simulink library "courseFollow_cl"  (R2018b)
settings: Solver=VariableStepAuto  StartTime=0.0  StopTime=10.0  RelTol=1e-3
undefined symbols (not defined in the file): a, initS, pathCtrl
libraries: angleBtw2Vecs_ul x3, vectorNormalizer_ul x3, schmehlTangentRotation_ul x1
settings Model: Creator=James Reed  LastModifiedBy=mcobb

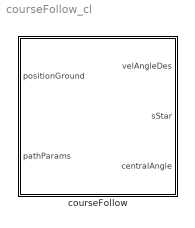
== system courseFollow_cl ==
  courseFollow : Subsystem

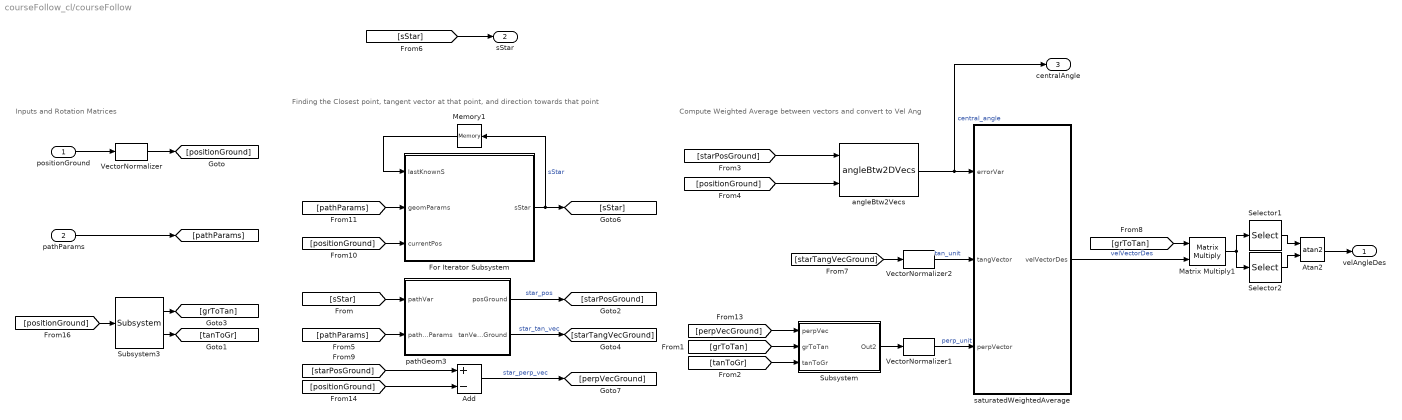
== system courseFollow_cl/courseFollow ==
  note: Compute Weighted Average between vectors and convert to Vel Ang
  note: Inputs and Rotation Matrices
  note: Finding the Closest point, tangent vector at that point, and direction towards that point
  "positionGround " : Inport
  pathParams : Inport  Port=2
  Add : Sum  Inputs=+-
  Atan2 : Trigonometry  Operator=atan2
  For Iterator Subsystem : Subsystem  TreatAsAtomicUnit=on
  Matrix Multiply1 : Product  Multiplication=Matrix(*)
  Memory1 : Memory  InitialCondition=initS
  Selector1 : Selector  InputPortWidth=3  IndexOptions=Index vector (dialog)  Indices=2  OutputSizes=1
  Selector2 : Selector  InputPortWidth=3  IndexOptions=Index vector (dialog)  Indices=1  OutputSizes=1
  Subsystem : Subsystem
  Subsystem3 : schmehlTangentRotation_ul/Subsystem  SystemSampleTime=-1
  "VectorNormalizer " : vectorNormalizer_ul/VectorNormalizer   SystemSampleTime=-1
  VectorNormalizer1 : vectorNormalizer_ul/VectorNormalizer   SystemSampleTime=-1
  VectorNormalizer2 : vectorNormalizer_ul/VectorNormalizer   SystemSampleTime=-1
  angleBtw2Vecs : angleBtw2Vecs_ul/angleBtw2DVecs  SystemSampleTime=-1
  pathGeom3 : MATLAB Function  TreatAsAtomicUnit=on
  saturatedWeightedAverage : Subsystem  mask{error_upper_lim=pathCtrl.perpErrorVal.Value}
      mask prompts: error_upper_lim "Value of Error yielding 100% perpendicular"
  velAngleDes : Outport
  sStar : Outport  Port=2
  centralAngle : Outport  Port=3
  wires:
  "VectorNormalizer "/1 -> [positionGround]
  [starPosGround] -> angleBtw2Vecs/1
  pathParams/1 -> [pathParams]
  VectorNormalizer2/1 -> saturatedWeightedAverage/2(tangVector)  "tan_unit"
  saturatedWeightedAverage/1("velVectorDes ") -> Matrix Multiply1/2  "velVectorDes"
  [positionGround] -> For Iterator Subsystem/3(currentPos)
  [positionGround] -> Subsystem3/1
  "positionGround "/1 -> "VectorNormalizer "/1
  Subsystem3/1 -> [grToTan]
  pathGeom3/1(posGround) -> [starPosGround]  "star_pos"
  [pathParams] -> pathGeom3/2(pathGeomParams)
  VectorNormalizer1/1 -> saturatedWeightedAverage/3("perpVector ")  "perp_unit"
  angleBtw2Vecs/1 -> centralAngle/1, saturatedWeightedAverage/1("errorVar ")  "central_angle"
  [positionGround] -> angleBtw2Vecs/2
  [sStar] -> pathGeom3/1(pathVar)
  [starTangVecGround] -> VectorNormalizer2/1
  [pathParams] -> For Iterator Subsystem/2(geomParams)
  Subsystem3/2 -> [tanToGr]
  [grToTan] -> Matrix Multiply1/1
  Matrix Multiply1/1 -> Selector2/1, Selector1/1
  Selector1/1 -> Atan2/1
  Selector2/1 -> Atan2/2
  Atan2/1 -> velAngleDes/1
  For Iterator Subsystem/1(sStar) -> [sStar], Memory1/1  "sStar"
  Memory1/1 -> For Iterator Subsystem/1(lastKnownS)
  Add/1 -> [perpVecGround]  "star_perp_vec"
  [positionGround] -> Add/2
  [starPosGround] -> Add/1
  pathGeom3/2(tanVecGround) -> [starTangVecGround]  "star_tan_vec"
  [perpVecGround] -> Subsystem/1(perpVec)
  Subsystem/1(Out2) -> VectorNormalizer1/1
  [grToTan] -> Subsystem/2(grToTan)
  [tanToGr] -> Subsystem/3(tanToGr)
  [sStar] -> sStar/1

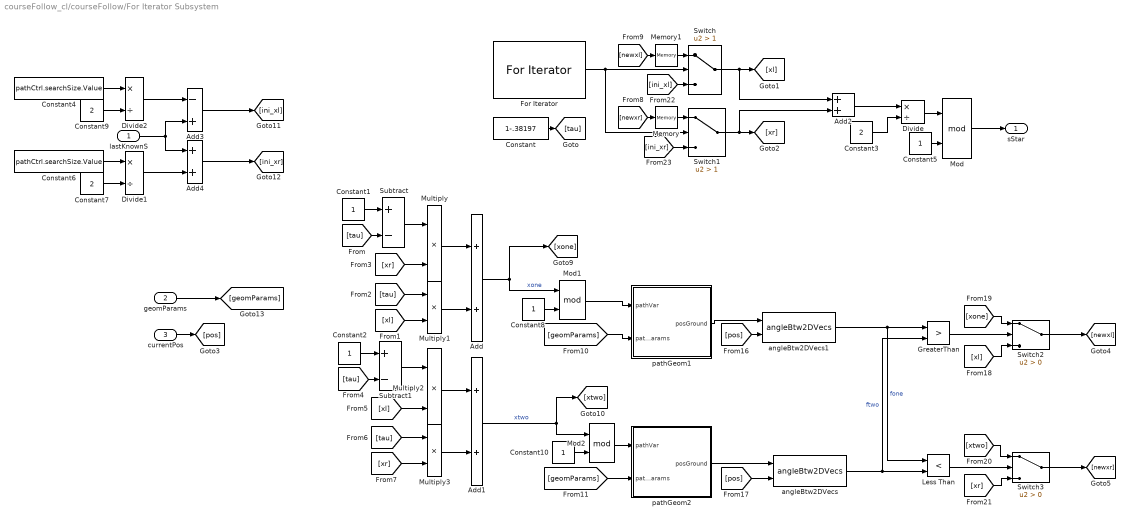
== system courseFollow_cl/courseFollow/For Iterator Subsystem ==
  lastKnownS : Inport
  geomParams : Inport  Port=2
  currentPos : Inport  Port=3
  Add{,1..2,4} (4 alike) : Sum
  Add3 : Sum  Inputs=-+
  Constant : Constant  Value=1-.38197
  Constant{1..2,5,8,10} (5 alike) : Constant
  Constant3 : Constant  Value=2
  Constant4 : Constant  Value=pathCtrl.searchSize.Value
  Constant6 : Constant  Value=pathCtrl.searchSize.Value
  Constant7 : Constant  Value=2
  Constant9 : Constant  Value=2
  Divide : Product  Inputs=*/
  Divide1 : Product  Inputs=*/
  Divide2 : Product  Inputs=*/
  For Iterator : ForIterator  IterationLimit=100
  GreaterThan : RelationalOperator  Operator=>  OutDataTypeStr=boolean  RndMeth=Simplest
  Less Than : RelationalOperator  Operator=<  OutDataTypeStr=boolean  RndMeth=Simplest
  Memory : Memory  InheritSampleTime=on
  Memory1 : Memory  InheritSampleTime=on
  Mod : Math  Operator=mod  SaturateOnIntegerOverflow=on
  Mod1 : Math  Operator=mod  SaturateOnIntegerOverflow=on
  Mod2 : Math  Operator=mod  SaturateOnIntegerOverflow=on
  Multiply{,1..3} (4 alike) : Product
  Subtract : Sum  Inputs=+-
  Subtract1 : Sum  Inputs=+-
  Switch : Switch  Criteria=u2 > Threshold  Threshold=1
  Switch1 : Switch  Criteria=u2 > Threshold  Threshold=1
  Switch2 : Switch  Criteria=u2 > Threshold
  Switch3 : Switch  Criteria=u2 > Threshold
  angleBtw2DVecs : angleBtw2Vecs_ul/angleBtw2DVecs  SystemSampleTime=-1
  angleBtw2DVecs1 : angleBtw2Vecs_ul/angleBtw2DVecs  SystemSampleTime=-1
  pathGeom1 : MATLAB Function  TreatAsAtomicUnit=on
  pathGeom2 : MATLAB Function  TreatAsAtomicUnit=on
  sStar : Outport
  wires:
  Constant3/1 -> Divide/2
  Add2/1 -> Divide/1
  Constant/1 -> [tau]
  Constant1/1 -> Subtract/1
  [tau] -> Subtract/2
  currentPos/1 -> [pos]
  Constant2/1 -> Subtract1/1
  [tau] -> Subtract1/2
  Subtract/1 -> Multiply/1
  [tau] -> Multiply3/1
  [xr] -> Multiply3/2
  [xl] -> Multiply2/2
  Subtract1/1 -> Multiply2/1
  Multiply/1 -> Add/1
  Multiply1/1 -> Add/2
  Multiply2/1 -> Add1/1
  Multiply3/1 -> Add1/2
  [tau] -> Multiply1/1
  [xl] -> Multiply1/2
  [xr] -> Multiply/2
  Switch/1 -> Add2/1, [xl]
  For Iterator/1 -> Switch1/2, Switch/2
  Switch1/1 -> Add2/2, [xr]
  Add/1 -> Mod1/1, [xone]  "xone"
  Add1/1 -> [xtwo], Mod2/1  "xtwo"
  geomParams/1 -> [geomParams]
  pathGeom1/1(posGround) -> angleBtw2DVecs1/1
  pathGeom2/1(posGround) -> angleBtw2DVecs/1
  [pos] -> angleBtw2DVecs1/2
  [pos] -> angleBtw2DVecs/2
  angleBtw2DVecs/1 -> GreaterThan/2, Less Than/2  "ftwo"
  angleBtw2DVecs1/1 -> Less Than/1, GreaterThan/1  "fone"
  GreaterThan/1 -> Switch2/2
  Less Than/1 -> Switch3/2
  Switch3/1 -> [newxr]
  Switch2/1 -> [newxl]
  [xl] -> Switch2/3
  [xone] -> Switch2/1
  [xtwo] -> Switch3/1
  [xr] -> Switch3/3
  [newxr] -> Memory/1
  Memory/1 -> Switch1/1
  [newxl] -> Memory1/1
  Memory1/1 -> Switch/1
  [ini_xl] -> Switch/3
  [ini_xr] -> Switch1/3
  lastKnownS/1 -> Add3/2, Add4/1
  Divide1/1 -> Add4/2
  [geomParams] -> pathGeom1/2(pathGeomParams)
  [geomParams] -> pathGeom2/2(pathGeomParams)
  Add4/1 -> [ini_xr]
  Add3/1 -> [ini_xl]
  Constant9/1 -> Divide2/2
  Constant4/1 -> Divide2/1
  Divide2/1 -> Add3/1
  Constant7/1 -> Divide1/2
  Constant6/1 -> Divide1/1
  Divide/1 -> Mod/1
  Constant5/1 -> Mod/2
  Mod/1 -> sStar/1
  Constant8/1 -> Mod1/2
  Mod1/1 -> pathGeom1/1(pathVar)
  Constant10/1 -> Mod2/2
  Mod2/1 -> pathGeom2/1(pathVar)

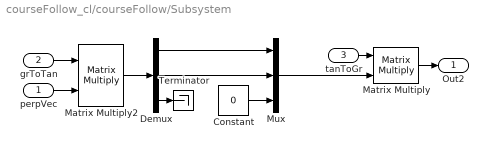
== system courseFollow_cl/courseFollow/Subsystem ==
  perpVec : Inport
  grToTan : Inport  Port=2
  tanToGr : Inport  Port=3
  Constant : Constant  Value=0
  Demux : Demux  Outputs=3
  Matrix Multiply : Product  Multiplication=Matrix(*)
  Matrix Multiply2 : Product  Multiplication=Matrix(*)
  Mux : Mux  Inputs=3
  Terminator : Terminator
  Out2 : Outport
  wires:
  Matrix Multiply2/1 -> Demux/1
  perpVec/1 -> Matrix Multiply2/2
  Constant/1 -> Mux/3
  Demux/1 -> Mux/1
  Demux/2 -> Mux/2
  Demux/3 -> Terminator/1
  Matrix Multiply/1 -> Out2/1
  Mux/1 -> Matrix Multiply/2
  tanToGr/1 -> Matrix Multiply/1
  grToTan/1 -> Matrix Multiply2/1

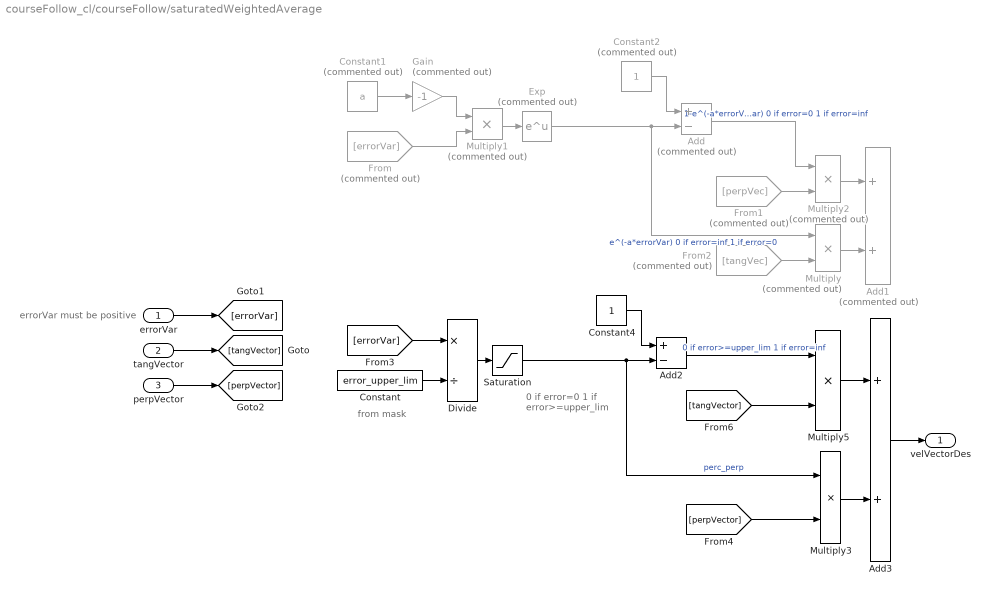
== system courseFollow_cl/courseFollow/saturatedWeightedAverage ==
  note: errorVar must be positive
  note: from mask
  note: 0 if error=0
      | 1 if error>=upper_lim
  "errorVar " : Inport
  tangVector : Inport  Port=2
  "perpVector " : Inport  Port=3
  Add : Sum  Commented=on  Inputs=+-
  Add1 : Sum  Commented=on
  Add2 : Sum  Inputs=+-
  Add3 : Sum
  Constant : Constant  Value=error_upper_lim
  Constant1 : Constant  Commented=on  Value=a
  Constant2 : Constant  Commented=on
  Constant4 : Constant
  Divide : Product  Inputs=*/
  Exp : Math  Commented=on  SaturateOnIntegerOverflow=on
  From : From  Commented=on  GotoTag=errorVar
  From1 : From  Commented=on  GotoTag=perpVec
  From2 : From  Commented=on  GotoTag=tangVec
  Gain : Gain  Commented=on  Gain=-1
  Multiply : Product  Commented=on
  Multiply1 : Product  Commented=on
  Multiply2 : Product  Commented=on
  Multiply3 : Product
  Multiply5 : Product
  Saturation : Saturate  UpperLimit=1  LowerLimit=0
  "velVectorDes " : Outport
  wires:
  [perpVector] -> Multiply3/2
  [tangVector] -> Multiply5/2
  Divide/1 -> Saturation/1
  Constant/1 -> Divide/2
  [errorVar] -> Divide/1
  Add2/1 -> Multiply5/1  "0 if error>=upper_lim 1 if error=inf"
  Multiply5/1 -> Add3/1
  Multiply3/1 -> Add3/2
  Add3/1 -> "velVectorDes "/1
  Saturation/1 -> Add2/2, Multiply3/1  "perc_perp"
  Constant4/1 -> Add2/1
  From2/1 -> Multiply/2
  From1/1 -> Multiply2/2
  Multiply/1 -> Add1/2
  Multiply2/1 -> Add1/1
  From/1 -> Multiply1/2
  "perpVector "/1 -> [perpVector]
  "errorVar "/1 -> [errorVar]
  Add/1 -> Multiply2/1  "1-e^(-a*errorVar) 0 if error=0 1 if error=inf"
  Constant2/1 -> Add/1
  Exp/1 -> Add/2, Multiply/1  "e^(-a*errorVar) 0 if error=inf 1 if error=0"
  Multiply1/1 -> Exp/1
  Gain/1 -> Multiply1/1
  Constant1/1 -> Gain/1
  tangVector/1 -> [tangVector]

== matlab function courseFollow_cl/courseFollow/For Iterator Subsystem/pathGeom1 ==
  data: pathVar input; posGround output; pathGeomParams input
function posGround = pathGeom1(pathVar, pathGeomParams)
    posGround = swapablePath(pathVar, pathGeomParams);
end

== matlab function courseFollow_cl/courseFollow/pathGeom3 ==
  data: pathVar input; posGround output; pathGeomParams input; tanVecGround output
function [posGround,tanVecGround] = pathGeom3(pathVar, pathGeomParams)
    [posGround,tanVecGround] = swapablePath(pathVar, pathGeomParams);
end

== matlab function courseFollow_cl/courseFollow/For Iterator Subsystem/pathGeom2 ==
  data: pathVar input; posGround output; pathGeomParams input
function posGround = pathGeom2(pathVar, pathGeomParams)
    posGround = swapablePath(pathVar, pathGeomParams);
end
